simulink library "csu_rgm_rtk_gps_meas_lib"  (R2014b)
settings: Solver=ode45  SolverMode=SingleTasking  StartTime=0.0  StopTime=10.0  RelTol=1e-3
values from neighbouring files (symbols this model uses):
  snp_rgm_index = [ 7 8 9 10 11 12 ]    [csc_snp_sensor_prep_mtv_init.m]
  snp_rgm_pos_only_index = [ 7 8 9 0 0 0]    [csc_snp_sensor_prep_mtv_init.m]
  snp_rgm_zero_index = [ 0 0 0 0 0 0]    [csc_snp_sensor_prep_mtv_init.m]
undefined symbols (not defined in the file or in its folder): kfl_use_gps_meas, kfl_use_gps_vel_meas
libraries: simulink x5, util_event_lib x2, util_info_lib x1, csu_und_unduplicate_lib x1, util_common_lib x1
settings Model: ExtModeAutoUpdateStatusClock=off  Creator=Administrator  LastModifiedBy=mstewart

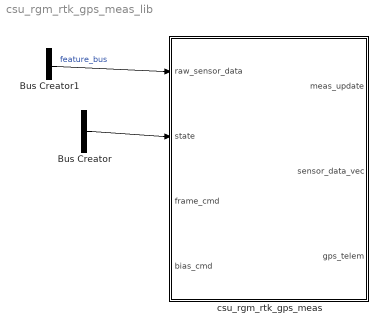
== system csu_rgm_rtk_gps_meas_lib ==
  Bus Creator : BusCreator
  Bus Creator1 : BusCreator  Inputs=2  OutDataTypeStr=Bus: feature_msg  NonVirtualBus=on
  csu_rgm_rtk_gps_meas : Subsystem
  wires:
  ? -> Bus Creator/2  "accel"
  ? -> Bus Creator/3  "rate"
  ? -> Bus Creator/1  "x"
  ? -> Bus Creator/4  "q"
  Bus Creator/1 -> csu_rgm_rtk_gps_meas/2(state)
  ? -> Bus Creator1/2  "pixels_2"
  ? -> Bus Creator1/1  "pixels_1"
  Bus Creator1/1 -> csu_rgm_rtk_gps_meas/1(raw_sensor_data)  "feature_bus"

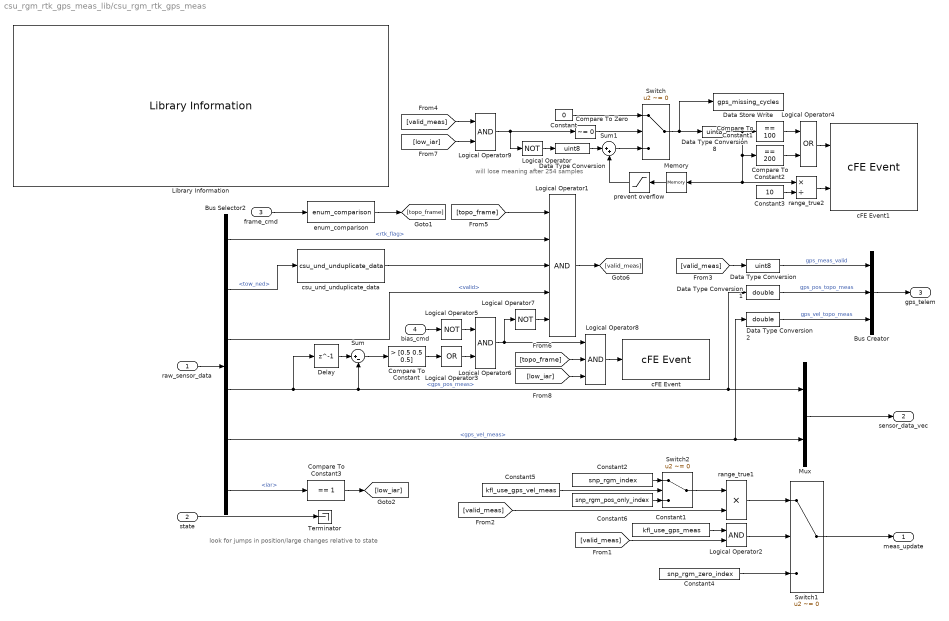
== system csu_rgm_rtk_gps_meas_lib/csu_rgm_rtk_gps_meas ==
  note: look for jumps in position/large changes relative to state
  note: will lose meaning after 254 samples
  raw_sensor_data : Inport
  state : Inport  Port=2
  frame_cmd : Inport  Port=3
  bias_cmd : Inport  Port=4
  Bus Creator : BusCreator  Inputs=3
  Bus Selector2 : BusSelector  OutputSignals=rtk_flag,tow_ned,valid,gps_pos_meas,gps_vel_meas,iar
  Compare To Constant : simulink/Logic and Bit Operations/Compare To Constant  relop=>  const=[0.5 0.5 0.5]  OutDataTypeStr=boolean
  Compare To Constant1 : simulink/Logic and Bit Operations/Compare To Constant  relop===  const=100  OutDataTypeStr=boolean
  Compare To Constant2 : simulink/Logic and Bit Operations/Compare To Constant  relop===  const=200  OutDataTypeStr=boolean
  Compare To Constant3 : simulink/Logic and Bit Operations/Compare To Constant  relop===  const=1  OutDataTypeStr=boolean
  Compare To Zero : simulink/Logic and Bit Operations/Compare To Zero  relop=~=  OutDataTypeStr=boolean
  Constant : Constant  Value=0  OutDataTypeStr=uint8
  Constant1 : Constant  Value=kfl_use_gps_meas
  Constant2 : Constant  Value=snp_rgm_index
  Constant3 : Constant  Value=10  OutDataTypeStr=uint8
  Constant4 : Constant  Value=snp_rgm_zero_index
  Constant5 : Constant  Value=kfl_use_gps_vel_meas
  Constant6 : Constant  Value=snp_rgm_pos_only_index
  Data Store Write : DataStoreWrite  DataStoreName=gps_missing_cycles
  Data Type Conversion : DataTypeConversion  OutDataTypeStr=uint8
  Data Type Conversion1 : DataTypeConversion  OutDataTypeStr=double
  Data Type Conversion2 : DataTypeConversion  OutDataTypeStr=double
  Data Type Conversion7 : DataTypeConversion  OutDataTypeStr=uint8
  Data Type Conversion8 : DataTypeConversion  OutDataTypeStr=uint8
  Delay : Delay  DelayLength=1  InitialCondition=0
  Library Information : util_info_lib/Library Information  owner='escrane'
  Logical Operator : Logic  Operator=NOT  AllPortsSameDT=off  OutDataTypeStr=boolean
  Logical Operator1 : Logic  Inputs=5  AllPortsSameDT=off  OutDataTypeStr=boolean
  Logical Operator2 : Logic  AllPortsSameDT=off  OutDataTypeStr=boolean
  Logical Operator3 : Logic  Operator=OR  Inputs=1  AllPortsSameDT=off  OutDataTypeStr=boolean
  Logical Operator4 : Logic  Operator=OR  AllPortsSameDT=off  OutDataTypeStr=boolean
  Logical Operator5 : Logic  Operator=NOT  Inputs=1  AllPortsSameDT=off  OutDataTypeStr=boolean
  Logical Operator6 : Logic  AllPortsSameDT=off  OutDataTypeStr=boolean
  Logical Operator7 : Logic  Operator=NOT  Inputs=1  AllPortsSameDT=off  OutDataTypeStr=boolean
  Logical Operator8 : Logic  Inputs=3  AllPortsSameDT=off  OutDataTypeStr=boolean
  Logical Operator9 : Logic  AllPortsSameDT=off  OutDataTypeStr=boolean
  Memory : Memory  X0=uint8(0)  InheritSampleTime=on
  Mux : Mux  Inputs=2
  Sum : Sum  Inputs=|+-
  Sum1 : Sum  Inputs=|++
  Switch : Switch  Criteria=u2 ~= 0
  Switch1 : Switch  Criteria=u2 ~= 0
  Switch2 : Switch  Criteria=u2 ~= 0
  Terminator : Terminator
  cFE Event : util_event_lib/cFE Event  event_message='GPS measurement has jumped--declaring invalid'  event_id=46  event_severity=INFORMATION  event_use_enums=off  event_enum_types={}
  cFE Event1 : util_event_lib/cFE Event  event_message='GPS NED measurement dropout for %i sec'  event_id=46  event_severity=INFORMATION  event_use_enums=off  event_enum_types={}
  csu_und_unduplicate_data : csu_und_unduplicate_lib/csu_und_unduplicate_data  initial_compare=0
  enum_comparison : util_common_lib/enum_comparison  comparison_type===
  prevent overflow : Saturate  UpperLimit=254  LowerLimit=0
  range_true1 : Product  RndMeth=Zero
  range_true2 : Product  Inputs=*/  RndMeth=Zero
  meas_update : Outport
  sensor_data_vec : Outport  Port=2
  gps_telem : Outport  Port=3
  wires:
  Data Type Conversion2/1 -> Bus Creator/3  "gps_vel_topo_meas"
  Switch2/1 -> range_true1/1
  Constant6/1 -> Switch2/3
  Constant5/1 -> Switch2/2
  Constant2/1 -> Switch2/1
  Mux/1 -> sensor_data_vec/1
  Bus Selector2/5 -> Mux/2, Data Type Conversion2/1  "<gps_vel_meas>"
  [low_iar] -> Logical Operator8/3
  [low_iar] -> Logical Operator9/2
  [valid_meas] -> Logical Operator9/1
  Compare To Constant3/1 -> [low_iar]
  Bus Selector2/6 -> Compare To Constant3/1  "<iar>"
  [topo_frame] -> Logical Operator8/2
  Logical Operator8/1 -> cFE Event/1
  enum_comparison/1 -> [topo_frame]
  [topo_frame] -> Logical Operator1/1
  Logical Operator7/1 -> Logical Operator1/5
  Logical Operator5/1 -> Logical Operator6/1
  Logical Operator3/1 -> Logical Operator6/2
  bias_cmd/1 -> Logical Operator5/1
  Bus Selector2/3 -> Logical Operator1/4  "<valid>"
  csu_und_unduplicate_data/1 -> Logical Operator1/3
  Bus Selector2/2 -> csu_und_unduplicate_data/1  "<tow_ned>"
  Data Type Conversion1/1 -> Bus Creator/2  "gps_pos_topo_meas"
  Data Type Conversion/1 -> Bus Creator/1  "gps_meas_valid"
  Bus Creator/1 -> gps_telem/1
  [valid_meas] -> Data Type Conversion/1
  Bus Selector2/1 -> Logical Operator1/2  "<rtk_flag>"
  [valid_meas] -> Logical Operator2/2
  Logical Operator2/1 -> Switch1/2
  Constant1/1 -> Logical Operator2/1
  range_true1/1 -> Switch1/1
  [valid_meas] -> range_true1/2
  frame_cmd/1 -> enum_comparison/1
  Bus Selector2/4 -> Delay/1, Sum/2, Mux/1, Data Type Conversion1/1  "<gps_pos_meas>"
  raw_sensor_data/1 -> Bus Selector2/1
  Switch1/1 -> meas_update/1
  Constant4/1 -> Switch1/3
  Logical Operator1/1 -> [valid_meas]
  state/1 -> Terminator/1
  Delay/1 -> Sum/1
  Sum/1 -> Compare To Constant/1
  Logical Operator9/1 -> Compare To Zero/1, Logical Operator/1
  Memory/1 -> prevent overflow/1
  Constant/1 -> Switch/1
  Sum1/1 -> Switch/3
  Compare To Zero/1 -> Switch/2
  Data Type Conversion7/1 -> Sum1/1
  Logical Operator/1 -> Data Type Conversion7/1
  prevent overflow/1 -> Sum1/2
  Switch/1 -> Data Type Conversion8/1, Data Store Write/1
  Data Type Conversion8/1 -> Compare To Constant1/1, Compare To Constant2/1, range_true2/1, Memory/1
  Compare To Constant/1 -> Logical Operator3/1
  Logical Operator6/1 -> Logical Operator8/1, Logical Operator7/1
  Compare To Constant1/1 -> Logical Operator4/1
  Compare To Constant2/1 -> Logical Operator4/2
  Logical Operator4/1 -> cFE Event1/1
  range_true2/1 -> cFE Event1/2
  Constant3/1 -> range_true2/2
